simulink library "lib_fuel_cell"  (Simulink 4.00)
undefined symbols (not defined in the file or in its folder): air_cp, amb_tmp, cell_const_F, cell_const_g, cell_const_jo, cell_const_LHV_H2, cell_const_Mair, cell_const_MH, cell_const_MW, cell_const_R2, cell_const_Voc, ex_gas_cp, fan_cool, fc_acc_mass, fc_act, fc_air_comp_map, fc_air_comp_pwr, fc_base_mass, fc_blower_rec_H2, fc_blowera, fc_c2i_th_cond, fc_c_init_tmp, fc_cell_area, fc_cell_const_eta1, fc_cell_const_eta_DCDC, fc_cell_const_etablow, fc_cell_const_etagen, fc_cell_const_etapump, fc_cell_const_ex, fc_cell_const_kw, fc_cell_const_Nrad, fc_cell_const_U, fc_cell_dim_A, fc_cell_dim_tm, fc_cell_num, fc_cell_press_a, fc_cell_press_amb, fc_cell_press_an, fc_cell_press_blowa, fc_cell_press_blowr, fc_cell_press_c, fc_cell_press_hum, fc_cell_press_hyd, fc_cell_stack_dpipe, fc_cell_stack_dpipefc, fc_cell_stack_drad, fc_cell_stack_Lpipe, fc_cell_stack_Lpipefc, fc_cell_stack_Lrad, fc_cell_stack_N, fc_cell_stack_Pel, fc_cell_stoich_RHah, fc_cell_stoich_RHch, fc_cell_stoich_RHo, fc_cell_stoich_vH, fc_cell_stoich_vO, fc_cell_stoich_XON, fc_cell_temp_ah, fc_cell_temp_amb, fc_cell_temp_cell ... (+74)
libraries: fc_vt_lib x2, lib_fuel_cell x1
(part 1 of 5)
settings Model: LastModifiedBy=kharalds

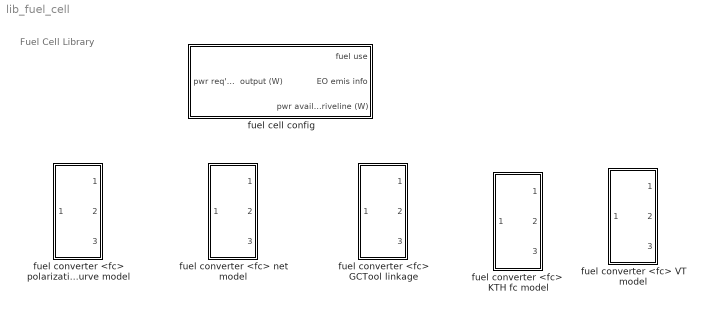
== system lib_fuel_cell ==
  note: Fuel Cell Library
  fuel cell config : Subsystem  BlockChoice=fuel converter <fc> net model
      settings: TemplateBlock=self  MemberBlocks="fuel converter <fc>  KTH fc model,fuel converter <fc> GCTool linkage,fuel converter <fc> VT model,fuel converter <fc> net model,fuel converter <fc> polarization curve model"  RTWFcnNameOpts=Auto  RTWFileNameOpts=Auto
  fuel converter <fc>  KTH fc model : Subsystem
      settings: RTWFcnNameOpts=Auto  RTWFileNameOpts=Auto
      mask Display: image(imread('bdi_fuelcell.jpg'))
  fuel converter <fc> GCTool linkage : Subsystem
      settings: RTWFcnNameOpts=Auto  RTWFileNameOpts=Auto
      mask Display: image(imread('bdi_fuelcell.jpg'))
  fuel converter <fc> VT model : Subsystem
      settings: RTWFcnNameOpts=Auto  RTWFileNameOpts=Auto
      mask Display: image(imread('bdi_fuelcell.jpg'))
  fuel converter <fc> net model : Subsystem
      settings: RTWFcnNameOpts=Auto  RTWFileNameOpts=Auto
      mask Display: image(imread('bdi_fuelcell.jpg'))
  fuel converter <fc> polarization curve model : Subsystem
      settings: RTWFcnNameOpts=Auto  RTWFileNameOpts=Auto
      mask Display: image(imread('bdi_fuelcell.jpg'))

== system lib_fuel_cell/fuel cell config ==
  pwr req'd at fc  output (W) : Inport  Port=1  LatchInput=off
  fuel converter <fc> net model : lib_fuel_cell/fuel converter <fc> net model
      link override fuel use and EO emis Fuel Cell/HOT engine maps /fuel (g//s): OutputValues=fc_fuel_map*fc_pwr_scale/fc_eff_scale
  fuel use : Outport  Port=1
  EO emis info : Outport  Port=2
  pwr avail. to driveline (W) : Outport  Port=3
  wires:
  pwr req'd at fc  output (W)/1 -> fuel converter <fc> net model/1
  fuel converter <fc> net model/1 -> fuel use/1
  fuel converter <fc> net model/2 -> EO emis info/1
  fuel converter <fc> net model/3 -> pwr avail. to driveline (W)/1

== system lib_fuel_cell/fuel converter <fc>  KTH fc model ==
  pwr req'd at fc  output (W) : Inport  Port=1  LatchInput=off
  Block NOTES : Subsystem
      settings: RTWFcnNameOpts=Auto  RTWFileNameOpts=Auto
      mask Display: disp('Block\nNOTES')
  Demux : Demux  Outputs=[1 4 1 1 1]  BusSelectionMode=off
  Demux1 : Demux  Outputs=[1 7 1]  BusSelectionMode=off
  Diagnostics : Subsystem
      settings: RTWFcnNameOpts=Auto  RTWFileNameOpts=Auto
  Mux1 : Mux  Inputs=7
  Temporary temperature : Constant  Value=[90 80 70 60]
  To Workspace2 : ToWorkspace  VariableName=fc_pwr_out_r  SampleTime=-1  SaveFormat=Array
  fuel cell  system <fc> : Subsystem
      settings: RTWFcnNameOpts=Auto  RTWFileNameOpts=Auto
  fuel use and EO emis Fuel Cell : Subsystem
      settings: RTWFcnNameOpts=Auto  RTWFileNameOpts=Auto
  fuel use : Outport  Port=1  InitialOutput=0
  EO emis info : Outport  Port=2  InitialOutput=0
  pwr avail. to driveline (W) : Outport  Port=3  InitialOutput=0
  tag scope: fc_pwr_out_a=global, fuel=global
  wires:
  fuel use and EO emis Fuel Cell/1(cum fuel  use (gal)) -> [fuel], fuel use/1
  fuel cell  system <fc>/1(power available (W) 1x1 emis info 7x1 fuel use 1x1) -> Demux1/1
  fuel use and EO emis Fuel Cell/3(Vv) -> Mux1/6
  fuel use and EO emis Fuel Cell/2("FC ON?, CO HC NOx PM mass flow exhaust exhaust temperature O2") -> Demux/1
  Demux1/1 -> pwr avail. to driveline (W)/1, [fc_pwr_out_a], fuel use and EO emis Fuel Cell/1(pwr (w))
  Demux1/2 -> fuel use and EO emis Fuel Cell/2(perf info)
  Demux1/3 -> fuel use and EO emis Fuel Cell/3(fuel use)
  pwr req'd at fc  output (W)/1 -> fuel cell  system <fc>/1(pwr req  (W)), To Workspace2/1
  fuel cell  system <fc>/2(system_characteristics) -> Diagnostics/1(In1)
  Temporary temperature/1 -> Mux1/7
  Mux1/1 -> EO emis info/1
  Demux/1 -> Mux1/1
  Demux/2 -> Mux1/2
  Demux/3 -> Mux1/3
  Demux/4 -> Mux1/4
  Demux/5 -> Mux1/5

== system lib_fuel_cell/fuel converter <fc> GCTool linkage ==
  pwr req'd at fc  output (W) : Inport  Port=1  LatchInput=off
  Block NOTES : Subsystem
      settings: RTWFcnNameOpts=Auto  RTWFileNameOpts=Auto
      mask Display: disp('Block\nNOTES')
  Constant : Constant  Value=fc_tstat
  Constant1 : Constant  Orientation=left  Value=0
  Constant3 : Constant  Value=fc_fuelcell_warmup_bool
  Constant4 : Constant  Orientation=left  Value=1
  Demux1 : Demux  Outputs=[1 7 1]  BusSelectionMode=off
  Mux : Mux  Inputs=2
      settings: DisplayOption=none
  Sum6 : Sum  Inputs=-+  SaturateOnIntegerOverflow=on
  Switch : Switch  Threshold=0
  Switch3 : Switch  Threshold=eps
  To Workspace2 : ToWorkspace  VariableName=fc_pwr_out_r  SampleTime=-1  SaveFormat=Array
  fuel cell  system <fc> : Subsystem
      settings: RTWFcnNameOpts=Auto  RTWFileNameOpts=Auto
  fuel use and EO emis Fuel Cell : Subsystem
      settings: RTWFcnNameOpts=Auto  RTWFileNameOpts=Auto
  gain : Gain  Gain=0.85  Multiplication=Element-wise(K.*u)  SaturateOnIntegerOverflow=on
  fuel use : Outport  Port=1  InitialOutput=0
  EO emis info : Outport  Port=2  InitialOutput=0
  pwr avail. to driveline (W) : Outport  Port=3  InitialOutput=0
  tag scope: fc_pwr_out_a=global, fuel=global
  wires:
  fuel use and EO emis Fuel Cell/1(cum fuel  use (gal)) -> [fuel], fuel use/1
  [coolant_temp] -> Sum6/2
  gain/1 -> Sum6/1
  Constant/1 -> gain/1
  Switch/1 -> [fc_pwr_out_a], pwr avail. to driveline (W)/1
  Switch3/1 -> Switch/2
  Sum6/1 -> Switch3/1
  Constant4/1 -> Switch3/3
  Constant3/1 -> Switch3/2
  Constant1/1 -> Switch/3
  pwr req'd at fc  output (W)/1 -> fuel cell  system <fc>/1(pwr req  (W)), To Workspace2/1
  fuel cell  system <fc>/1(power available (W) 1x1 emis info 7x1 fuel use 1x1) -> Demux1/1
  fuel use and EO emis Fuel Cell/3(Vv,Tfc) -> Mux/2
  fuel use and EO emis Fuel Cell/2("FC ON?, EOem, MFex, Tex, O2ex") -> Mux/1
  Mux/1 -> EO emis info/1
  Demux1/1 -> fuel use and EO emis Fuel Cell/1(pwr (w)), Switch/1
  Demux1/2 -> fuel use and EO emis Fuel Cell/2(perf info)
  Demux1/3 -> fuel use and EO emis Fuel Cell/3(fuel use)

== system lib_fuel_cell/fuel converter <fc> VT model ==
  note: May need to add enabled subsystem to top level (tm:8/12/02)
  pwr req'd at fc  output (W) : Inport  Port=1  LatchInput=off
  Block NOTES : Subsystem
      settings: RTWFcnNameOpts=Auto  RTWFileNameOpts=Auto
      mask Display: disp('Block\nNOTES')
  Fuel Cell Power System Model (S. Gurski - Virgina Tech) : Subsystem
      settings: RTWFcnNameOpts=Auto  RTWFileNameOpts=Auto
  Mux : Mux  Inputs=2
      settings: DisplayOption=none
  To Workspace2 : ToWorkspace  VariableName=fc_pwr_out_r  SampleTime=-1  SaveFormat=Array
  diagnostics : Subsystem
      settings: RTWFcnNameOpts=Auto  RTWFileNameOpts=Auto
  fuel use and EO emis Fuel Cell : Subsystem
      settings: RTWFcnNameOpts=Auto  RTWFileNameOpts=Auto
  fuel use : Outport  Port=1  InitialOutput=0
  EO emis info : Outport  Port=2  InitialOutput=0
  pwr avail. to driveline (W) : Outport  Port=3  InitialOutput=0
  tag scope: fc_pwr_out_a=global, fuel=global
  wires:
  Mux/1 -> EO emis info/1
  fuel use and EO emis Fuel Cell/2("FC ON?, EOem, MFex, Tex, O2ex") -> Mux/1
  fuel use and EO emis Fuel Cell/3(Vv,Tfc) -> Mux/2
  Fuel Cell Power System Model (S. Gurski - Virgina Tech)/1(Net Power Gen) -> fuel use and EO emis Fuel Cell/1(pwr (w)), pwr avail. to driveline (W)/1, [fc_pwr_out_a]
  pwr req'd at fc  output (W)/1 -> To Workspace2/1, Fuel Cell Power System Model (S. Gurski - Virgina Tech)/1(Net Power Request)
  fuel use and EO emis Fuel Cell/1(cum fuel  use (gal)) -> fuel use/1, [fuel]
  Fuel Cell Power System Model (S. Gurski - Virgina Tech)/2(system_characteristics) -> fuel use and EO emis Fuel Cell/2(system info), diagnostics/1(In1)

== system lib_fuel_cell/fuel converter <fc> net model ==
  pwr req'd at fc  output (W) : Inport  Port=1  LatchInput=off
  Block NOTES : Subsystem
      settings: RTWFcnNameOpts=Auto  RTWFileNameOpts=Auto
      mask Display: disp('Block\nNOTES')
  Constant : Constant  Value=fc_tstat
  Constant1 : Constant  Orientation=left  Value=0
  Constant3 : Constant  Value=fc_fuelcell_warmup_bool
  Constant4 : Constant  Orientation=left  Value=1
  Mux : Mux  Inputs=2
      settings: DisplayOption=none
  Sum6 : Sum  Inputs=-+  SaturateOnIntegerOverflow=on
  Switch : Switch  Threshold=0
  Switch3 : Switch  Threshold=eps
  To Workspace2 : ToWorkspace  VariableName=fc_pwr_out_r  SampleTime=-1  SaveFormat=Array
  fuel cell  system <fc> : Subsystem
      settings: RTWFcnNameOpts=Auto  RTWFileNameOpts=Auto
  fuel use and EO emis Fuel Cell : Subsystem
      settings: RTWFcnNameOpts=Auto  RTWFileNameOpts=Auto
  gain : Gain  Gain=0.85  Multiplication=Element-wise(K.*u)  SaturateOnIntegerOverflow=on
  fuel use : Outport  Port=1  InitialOutput=0
  EO emis info : Outport  Port=2  InitialOutput=0
  pwr avail. to driveline (W) : Outport  Port=3  InitialOutput=0
  tag scope: fc_pwr_out_a=global, fuel=global
  wires:
  Mux/1 -> EO emis info/1
  fuel use and EO emis Fuel Cell/2("FC ON?, EOem, MFex, Tex, O2ex") -> Mux/1
  fuel use and EO emis Fuel Cell/3(Vv,Tfc) -> Mux/2
  fuel cell  system <fc>/1(power available (W) 1x1) -> fuel use and EO emis Fuel Cell/1(pwr (w)), Switch/1
  pwr req'd at fc  output (W)/1 -> To Workspace2/1, fuel cell  system <fc>/1(pwr req  (W))
  Constant1/1 -> Switch/3
  Constant3/1 -> Switch3/2
  Constant4/1 -> Switch3/3
  Sum6/1 -> Switch3/1
  Switch3/1 -> Switch/2
  Switch/1 -> pwr avail. to driveline (W)/1, [fc_pwr_out_a]
  Constant/1 -> gain/1
  gain/1 -> Sum6/1
  [coolant_temp] -> Sum6/2
  fuel use and EO emis Fuel Cell/1(cum fuel  use (gal)) -> fuel use/1, [fuel]

== system lib_fuel_cell/fuel converter <fc> polarization curve model ==
  pwr req'd at fc  output (W) : Inport  Port=1  LatchInput=off
  Block NOTES : Subsystem
      settings: RTWFcnNameOpts=Auto  RTWFileNameOpts=Auto
      mask Display: disp('Block\nNOTES')
  Constant : Constant  Value=fc_tstat
  Constant1 : Constant  Orientation=left  Value=0
  Constant3 : Constant  Value=fc_fuelcell_warmup_bool
  Constant4 : Constant  Orientation=left  Value=1
  Demux1 : Demux  Outputs=[1 1 6 1 1]  BusSelectionMode=off
  Mux : Mux  Inputs=2
      settings: DisplayOption=none
  Sum6 : Sum  Inputs=-+  SaturateOnIntegerOverflow=on
  Switch : Switch  Threshold=0
  Switch3 : Switch  Threshold=eps
  To Workspace2 : ToWorkspace  VariableName=fc_pwr_out_r  SampleTime=-1  SaveFormat=Array
  fuel cell  system <fc> : Subsystem
      settings: RTWFcnNameOpts=Auto  RTWFileNameOpts=Auto
  fuel use and EO emis Fuel Cell : Subsystem
      settings: RTWFcnNameOpts=Auto  RTWFileNameOpts=Auto
  gain : Gain  Gain=0.85  Multiplication=Element-wise(K.*u)  SaturateOnIntegerOverflow=on
  fuel use : Outport  Port=1  InitialOutput=0
  EO emis info : Outport  Port=2  InitialOutput=0
  pwr avail. to driveline (W) : Outport  Port=3  InitialOutput=0
  tag scope: fc_pwr_out_a=global, fuel=global
  wires:
  fuel use and EO emis Fuel Cell/1(cum fuel  use (gal)) -> [fuel], fuel use/1
  [coolant_temp] -> Sum6/2
  gain/1 -> Sum6/1
  Constant/1 -> gain/1
  Switch/1 -> [fc_pwr_out_a], pwr avail. to driveline (W)/1
  Switch3/1 -> Switch/2
  Sum6/1 -> Switch3/1
  Constant4/1 -> Switch3/3
  Constant3/1 -> Switch3/2
  Constant1/1 -> Switch/3
  pwr req'd at fc  output (W)/1 -> fuel cell  system <fc>/1(pwr req  (W)), To Workspace2/1
  fuel cell  system <fc>/1(power net (W) 1x1 power gross (W) 1x1 emis info 6x1 fuel use 1x1 Texh 1x1) -> Demux1/1
  fuel use and EO emis Fuel Cell/3(Vv,Tfc) -> Mux/2
  fuel use and EO emis Fuel Cell/2("FC ON?, EOem, MFex, Tex, O2ex") -> Mux/1
  Mux/1 -> EO emis info/1
  Demux1/5 -> fuel use and EO emis Fuel Cell/5(Texh)
  Demux1/4 -> fuel use and EO emis Fuel Cell/4(fuel use)
  Demux1/3 -> fuel use and EO emis Fuel Cell/3(perf info)
  Demux1/1 -> fuel use and EO emis Fuel Cell/1(pwr net(w)), Switch/1
  Demux1/2 -> fuel use and EO emis Fuel Cell/2(pwr gross(w)1)

== system lib_fuel_cell/fuel converter <fc>  KTH fc model/Block NOTES ==
  note: This block models the internal combustion engine, and includes inertia effects,
      | performance limits, accessory loads, and temperature transient effects on fuel
      | use, engine-out emissions, and catalyst efficiency.  There are 'leads' to the
      | engine controller here, which controller determines whether the engine is on.

== system lib_fuel_cell/fuel converter <fc>  KTH fc model/Diagnostics ==
  In1 : Inport  Port=1  LatchInput=off
  Demux : Demux  Outputs=22  BusSelectionMode=off
  Terminator : Terminator
  Terminator1 : Terminator
  Terminator2 : Terminator
  To Workspace : ToWorkspace  VariableName=fc_net_pwr_req  SampleTime=-1  SaveFormat=Array
  To Workspace1 : ToWorkspace  VariableName=fc_net_pwr_gen  SampleTime=-1  SaveFormat=Array
  To Workspace10 : ToWorkspace  VariableName=fc_eta_fcsyst  SampleTime=-1  SaveFormat=Array
  To Workspace11 : ToWorkspace  VariableName=fc_gross_pwr  SampleTime=-1  SaveFormat=Array
  To Workspace13 : ToWorkspace  VariableName=fc_mdot_air  SampleTime=-1  SaveFormat=Array
  To Workspace14 : ToWorkspace  VariableName=w  SampleTime=-1  SaveFormat=Array
  To Workspace15 : ToWorkspace  VariableName=Qwc  SampleTime=-1  SaveFormat=Array
  To Workspace16 : ToWorkspace  VariableName=Qwa  SampleTime=-1  SaveFormat=Array
  To Workspace17 : ToWorkspace  VariableName=diff  SampleTime=-1  SaveFormat=Array
  To Workspace18 : ToWorkspace  VariableName=Qwtot  SampleTime=-1  SaveFormat=Array
  To Workspace19 : ToWorkspace  VariableName=Qevapc  SampleTime=-1  SaveFormat=Array
  To Workspace2 : ToWorkspace  VariableName=fc_auxiliary_pwr  SampleTime=-1  SaveFormat=Array
  To Workspace20 : ToWorkspace  VariableName=Qevapa  SampleTime=-1  SaveFormat=Array
  To Workspace21 : ToWorkspace  VariableName=Qhum  SampleTime=-1  SaveFormat=Array
  To Workspace3 : ToWorkspace  VariableName=fc_mdot_w_condc  SampleTime=-1  SaveFormat=Array
  To Workspace4 : ToWorkspace  VariableName=fc_current_density  SampleTime=-1  SaveFormat=Array
  To Workspace5 : ToWorkspace  VariableName=fc_mdot_H  SampleTime=-1  SaveFormat=Array
  To Workspace6 : ToWorkspace  VariableName=fc_mdot_w_conda  SampleTime=-1  SaveFormat=Array
  To Workspace9 : ToWorkspace  VariableName=fc_pwr_compressor  SampleTime=-1  SaveFormat=Array
  wires:
  In1/1 -> Demux/1
  Demux/1 -> To Workspace/1
  Demux/2 -> To Workspace1/1
  Demux/3 -> To Workspace2/1
  Demux/4 -> To Workspace3/1
  Demux/5 -> To Workspace4/1
  Demux/6 -> To Workspace5/1
  Demux/8 -> Terminator2/1
  Demux/10 -> To Workspace9/1
  Demux/11 -> To Workspace10/1
  Demux/12 -> To Workspace11/1
  Demux/13 -> Terminator1/1
  Demux/14 -> To Workspace13/1
  Demux/15 -> To Workspace14/1
  Demux/7 -> To Workspace6/1
  Demux/22 -> To Workspace21/1
  Demux/21 -> To Workspace20/1
  Demux/20 -> To Workspace19/1
  Demux/19 -> To Workspace18/1
  Demux/18 -> To Workspace16/1
  Demux/17 -> To Workspace15/1
  Demux/16 -> To Workspace17/1
  Demux/9 -> Terminator/1

== system lib_fuel_cell/fuel converter <fc>  KTH fc model/fuel cell  system <fc> ==
  pwr req  (W) : Inport  Port=1  LatchInput=off
  Block NOTES : Subsystem
      settings: RTWFcnNameOpts=Auto  RTWFileNameOpts=Auto
      mask Display: disp('Block\nNOTES')
  KTH fc model : Subsystem  TreatAsAtomicUnit=on
      settings: RTWFcnNameOpts=Auto  RTWFileNameOpts=Auto
  Mux2 : Mux  Inputs=[1 7 1]
      settings: DisplayOption=none
  power available (W) 1x1 emis info 7x1 fuel use 1x1 : Outport  Port=1  InitialOutput=0
  system_characteristics : Outport  Port=2  InitialOutput=0
  wires:
  [engine_on] -> KTH fc model/Enable
  Mux2/1 -> power available (W) 1x1 emis info 7x1 fuel use 1x1/1
  pwr req  (W)/1 -> KTH fc model/1(In1)
  KTH fc model/1(pwr avail. to driveline (W)) -> Mux2/1
  KTH fc model/2(Emissions info) -> Mux2/2
  KTH fc model/3(fuel use) -> Mux2/3
  KTH fc model/4(system characteristics) -> system_characteristics/1

== system lib_fuel_cell/fuel converter <fc>  KTH fc model/fuel use and EO emis Fuel Cell ==
  pwr (w) : Inport  Port=1  LatchInput=off
  perf info : Inport  Port=2  LatchInput=off
  fuel use : Inport  Port=3  LatchInput=off
  Block NOTES : Subsystem
      settings: RTWFcnNameOpts=Auto  RTWFileNameOpts=Auto
      mask Display: disp('Block\nNOTES')
  Demux1 : Demux  Outputs=7  BusSelectionMode=off
  Integrator : Integrator  ExternalReset=none  InitialConditionSource=internal  InitialCondition=0  LimitOutput=off  UpperSaturationLimit=inf  LowerSaturationLimit=-inf  ShowSaturationPort=off  ShowStatePort=off  AbsoluteTolerance=auto
  Mux1 : Mux  Inputs=4
      settings: DisplayOption=none
  Mux4 : Mux  Inputs=[1 4 1 1 1]
      settings: DisplayOption=none
  Terminator1 : Terminator
  To Workspace15 : ToWorkspace  VariableName=fc_fuel_rate  SampleTime=-1  SaveFormat=Array
  To Workspace8 : ToWorkspace  VariableName=fc_emis_eo  SampleTime=-1  SaveFormat=Array
  g/s-->gal/s : Gain  Gain=1/fc_fuel_den*61.02/231  Multiplication=Element-wise(K.*u)  SaturateOnIntegerOverflow=on
  cum fuel  use (gal) : Outport  Port=1  InitialOutput=0
  "FC ON?, CO HC NOx PM mass flow exhaust exhaust temperature O2" : Outport  Port=2  InitialOutput=0
  Vv : Outport  Port=3  InitialOutput=0
  wires:
  Demux1/7 -> Mux4/5
  Mux1/1 -> To Workspace8/1, Mux4/2
  g/s-->gal/s/1 -> Integrator/1
  Integrator/1 -> cum fuel  use (gal)/1
  Demux1/5 -> Mux4/3
  Demux1/6 -> Mux4/4
  pwr (w)/1 -> Terminator1/1
  perf info/1 -> Demux1/1
  Demux1/1 -> Mux1/1
  Demux1/2 -> Mux1/2
  Demux1/3 -> Mux1/3
  Demux1/4 -> Mux1/4
  fuel use/1 -> g/s-->gal/s/1, To Workspace15/1
  [v_prev] -> Vv/1
  [engine_on] -> Mux4/1
  Mux4/1 -> "FC ON?, CO HC NOx PM mass flow exhaust exhaust temperature O2"/1

== system lib_fuel_cell/fuel converter <fc> GCTool linkage/Block NOTES ==
  note: This block models the internal combustion engine, and includes inertia effects,
      | performance limits, accessory loads, and temperature transient effects on fuel
      | use, engine-out emissions, and catalyst efficiency.  There are 'leads' to the
      | engine controller here, which controller determines whether the engine is on.

== system lib_fuel_cell/fuel converter <fc> GCTool linkage/fuel cell  system <fc> ==
  pwr req  (W) : Inport  Port=1  LatchInput=off
  Block NOTES : Subsystem
      settings: RTWFcnNameOpts=Auto  RTWFileNameOpts=Auto
      mask Display: disp('Block\nNOTES')
  GCTool fuel cell model : Subsystem  TreatAsAtomicUnit=on
      settings: RTWFcnNameOpts=Auto  RTWFileNameOpts=Auto
  Mux2 : Mux  Inputs=[1 7 1]
      settings: DisplayOption=none
  power available (W) 1x1 emis info 7x1 fuel use 1x1 : Outport  Port=1  InitialOutput=0
  wires:
  pwr req  (W)/1 -> GCTool fuel cell model/1(net pwr req (W))
  Mux2/1 -> power available (W) 1x1 emis info 7x1 fuel use 1x1/1
  [engine_on] -> GCTool fuel cell model/Enable
  GCTool fuel cell model/1(net pwr out (W)) -> Mux2/1
  GCTool fuel cell model/2(emis info hc co nox pm MFexh Texh O2) -> Mux2/2
  GCTool fuel cell model/3(fuel use) -> Mux2/3

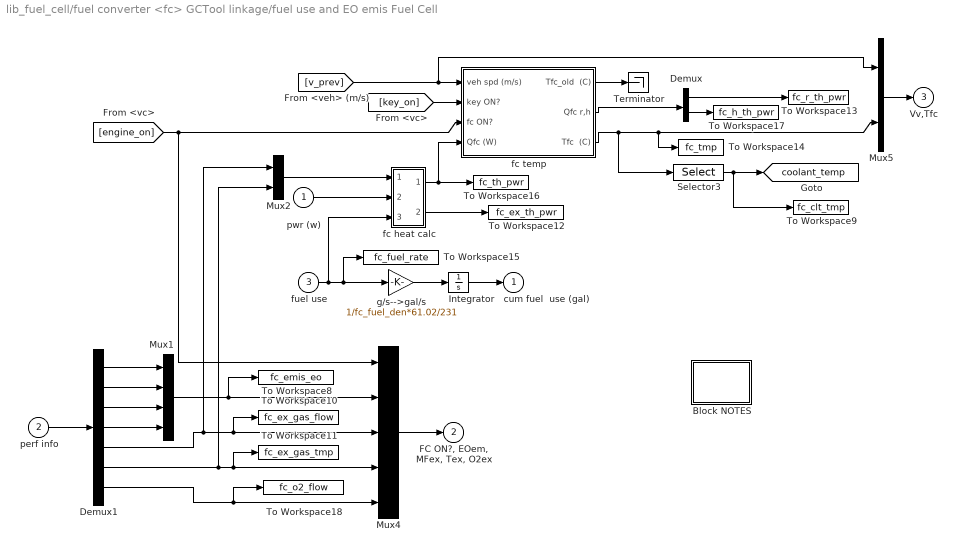
== system lib_fuel_cell/fuel converter <fc> GCTool linkage/fuel use and EO emis Fuel Cell ==
  pwr (w) : Inport  Port=1  LatchInput=off
  perf info : Inport  Port=2  LatchInput=off
  fuel use : Inport  Port=3  LatchInput=off
  Block NOTES : Subsystem
      settings: RTWFcnNameOpts=Auto  RTWFileNameOpts=Auto
      mask Display: disp('Block\nNOTES')
  Demux : Demux  Outputs=2  BusSelectionMode=off
  Demux1 : Demux  Outputs=7  BusSelectionMode=off
  Integrator : Integrator  ExternalReset=none  InitialConditionSource=internal  InitialCondition=0  LimitOutput=off  UpperSaturationLimit=inf  LowerSaturationLimit=-inf  ShowSaturationPort=off  ShowStatePort=off  AbsoluteTolerance=auto
  Mux1 : Mux  Inputs=4
      settings: DisplayOption=none
  Mux2 : Mux  Inputs=2
      settings: DisplayOption=none
  Mux4 : Mux  Inputs=[1 4 1 1 1]
      settings: DisplayOption=none
  Mux5 : Mux  Inputs=[1 4 ]
      settings: DisplayOption=none
  Selector3 : Selector  InputType=Vector  ElementSrc=Internal  Elements=2  RowSrc=Internal  Rows=1  ColumnSrc=Internal  Columns=1  InputPortWidth=4
  Terminator : Terminator
  To Workspace10 : ToWorkspace  VariableName=fc_ex_gas_flow  SampleTime=-1  SaveFormat=Array
  To Workspace11 : ToWorkspace  VariableName=fc_ex_gas_tmp  SampleTime=-1  SaveFormat=Array
  To Workspace12 : ToWorkspace  VariableName=fc_ex_th_pwr  SampleTime=-1  SaveFormat=Array
  To Workspace13 : ToWorkspace  VariableName=fc_r_th_pwr  SampleTime=-1  SaveFormat=Array
  To Workspace14 : ToWorkspace  VariableName=fc_tmp  SampleTime=-1  SaveFormat=Array
  To Workspace15 : ToWorkspace  VariableName=fc_fuel_rate  SampleTime=-1  SaveFormat=Array
  To Workspace16 : ToWorkspace  VariableName=fc_th_pwr  SampleTime=-1  SaveFormat=Array
  To Workspace17 : ToWorkspace  VariableName=fc_h_th_pwr  SampleTime=-1  SaveFormat=Array
  To Workspace18 : ToWorkspace  VariableName=fc_o2_flow  SampleTime=-1  SaveFormat=Array
  To Workspace8 : ToWorkspace  VariableName=fc_emis_eo  SampleTime=-1  SaveFormat=Array
  To Workspace9 : ToWorkspace  VariableName=fc_clt_tmp  SampleTime=-1  SaveFormat=Array
  fc heat calc : Subsystem
      settings: RTWFcnNameOpts=Auto  RTWFileNameOpts=Auto
  fc temp : Subsystem
      settings: RTWFcnNameOpts=Auto  RTWFileNameOpts=Auto
  g/s-->gal/s : Gain  Gain=1/fc_fuel_den*61.02/231  Multiplication=Element-wise(K.*u)  SaturateOnIntegerOverflow=on
  cum fuel  use (gal) : Outport  Port=1  InitialOutput=0
  "FC ON?, EOem, MFex, Tex, O2ex" : Outport  Port=2  InitialOutput=0
  Vv,Tfc : Outport  Port=3  InitialOutput=0
  tag scope: coolant_temp=global
  wires:
  Demux1/7 -> To Workspace18/1, Mux4/5
  Mux1/1 -> To Workspace8/1, Mux4/2
  g/s-->gal/s/1 -> Integrator/1
  Selector3/1 -> [coolant_temp], To Workspace9/1
  [engine_on] -> fc temp/3(fc ON?), Mux4/1
  Integrator/1 -> cum fuel  use (gal)/1
  Mux4/1 -> "FC ON?, EOem, MFex, Tex, O2ex"/1
  Demux1/5 -> To Workspace10/1, Mux4/3, Mux2/1
  Demux1/6 -> Mux4/4, To Workspace11/1, Mux2/2
  [key_on] -> fc temp/2(key ON?)
  Demux/2 -> To Workspace17/1
  Demux/1 -> To Workspace13/1
  fc temp/2(Qfc r,h) -> Demux/1
  fc temp/1(Tfc_old  (C)) -> Terminator/1
  fc temp/3(Tfc  (C)) -> Mux5/2, To Workspace14/1, Selector3/1
  [v_prev] -> fc temp/1(veh spd (m/s)), Mux5/1
  Mux5/1 -> Vv,Tfc/1
  pwr (w)/1 -> fc heat calc/2(In3)
  fc heat calc/2(Out1) -> To Workspace12/1
  perf info/1 -> Demux1/1
  Demux1/1 -> Mux1/1
  Demux1/2 -> Mux1/2
  Demux1/3 -> Mux1/3
  Demux1/4 -> Mux1/4
  Mux2/1 -> fc heat calc/1(In5)
  fc heat calc/1(Out2) -> fc temp/4(Qfc (W)), To Workspace16/1
  fuel use/1 -> g/s-->gal/s/1, To Workspace15/1, fc heat calc/3(In4)

== system lib_fuel_cell/fuel converter <fc> VT model/Block NOTES ==
  note: No block notes at this time.

== system lib_fuel_cell/fuel converter <fc> VT model/Fuel Cell Power System Model (S. Gurski - Virgina Tech) ==
  Net Power Request : Inport  Orientation=left  Port=1  LatchInput=off
  Algebraic Constraint1 : Subsystem  AncestorBlock=simulink3/Math/Algebraic Constraint  mask(Algebraic Constraint){z0=0.6}
      mask prompts: z0 "Initial guess:"
      mask help: Constrains input signal f(z) to zero and outputs an algebraic state z. This block outputs the value necessary to produce a zero at the input. The output must affect the input through some feedback path. Provide an initial guess of the output to improve algebraic loop solver efficiency.
      settings: RTWFcnNameOpts=Auto  RTWFileNameOpts=Auto
      mask Help:
      | This block outputs the value necessary to produce a zero at the input. The output must affect the input through some feedback path. This allows you to specify algebraic equations for index 1 differential/algebraic systems (DAE's).
      | 
      | By default, the initial guess is zero.  You can improve the efficiency of the algebraic loop solver by providing an initial guess that is close to the solution value.
      mask Display: disp('Solve\nf(z) = 0')
  Bus Creator : Subsystem
      settings: RTWFcnNameOpts=Auto  RTWFileNameOpts=Auto
  Constant1 : Constant  Value=fc_min_cell_volts
  Demux : Demux  Outputs=6  BusSelectionMode=off
  Demux1 : Demux  Outputs=6  BusSelectionMode=off
  Fuel Cell System : Subsystem  TreatAsAtomicUnit=on
      settings: RTWFcnNameOpts=Auto  RTWFileNameOpts=Auto
  Fuel Cell System - min voltage : Subsystem
      settings: RTWFcnNameOpts=Auto  RTWFileNameOpts=Auto
  If : If  NumInputs=2  IfExpression=u1 < u2  ShowElse=off
  Mux1 : Mux  Inputs=6
  Mux2 : Mux  Orientation=left  Inputs=6
  Sum2 : Sum  Inputs=|+-  SaturateOnIntegerOverflow=on
  Switch1 : Switch  Threshold=1
  Terminator : Terminator
  Water : Memory  Orientation=left  X0=0  InheritSampleTime=off
      settings: RTWStateStorageClass=Auto
  stack_temperature : Memory  Orientation=left  X0=fc_system_init_temp  InheritSampleTime=off
      settings: RTWStateStorageClass=Auto
  t_stack_coolant_in : Memory  Orientation=left  X0=fc_system_init_temp  InheritSampleTime=off
      settings: RTWStateStorageClass=Auto
  Net Power Gen : Outport  Port=1
  system_characteristics : Outport  Port=2
  wires:
  Demux/1 -> Net Power Gen/1
  Demux/2 -> stack_temperature/1
  Demux/4 -> t_stack_coolant_in/1
  Demux/5 -> Water/1
  t_stack_coolant_in/1 -> Mux2/2
  stack_temperature/1 -> Mux2/3
  Water/1 -> Mux2/4
  Bus Creator/1(system_characteristics) -> system_characteristics/1
  Demux/6 -> Bus Creator/1(In1)
  Net Power Request/1 -> Mux2/1
  Mux2/1 -> Demux1/1, Fuel Cell System/1(In1)
  Demux/3 -> Terminator/1
  [elevation] -> Mux2/5
  Constant1/1 -> Sum2/1
  Sum2/1 -> Algebraic Constraint1/1(f(z))
  Algebraic Constraint1/1(z) -> Fuel Cell System - min voltage/1(" Current Density Request")
  Fuel Cell System - min voltage/1(Net Power Gen) -> Mux1/1, If/2
  Fuel Cell System - min voltage/2(Stack Temperature) -> Mux1/2
  Fuel Cell System - min voltage/3(cell_voltage) -> Sum2/2, Mux1/3
  Fuel Cell System - min voltage/4(t_stack_coolant_in) -> Mux1/4
  Fuel Cell System - min voltage/5(waterbalance) -> Mux1/5
  Demux1/2 -> Fuel Cell System - min voltage/2(t_stack_coolant_in1)
  Demux1/3 -> Fuel Cell System - min voltage/3(fc_stack_temperature)
  Demux1/4 -> Fuel Cell System - min voltage/4(water_balance_previous)
  Demux1/1 -> If/1
  If/1 -> Fuel Cell System/Action
  Fuel Cell System/1(Out1) -> Switch1/1
  Fuel Cell System/2(Out2) -> Switch1/2
  Mux1/1 -> Switch1/3
  Fuel Cell System - min voltage/6(system_characteristics) -> Mux1/6
  Demux1/5 -> Fuel Cell System - min voltage/5(elevation)
  Switch1/1 -> Demux/1
  [v_prev] -> Mux2/6
  Demux1/6 -> Fuel Cell System - min voltage/6(vehicle speed (m/s))

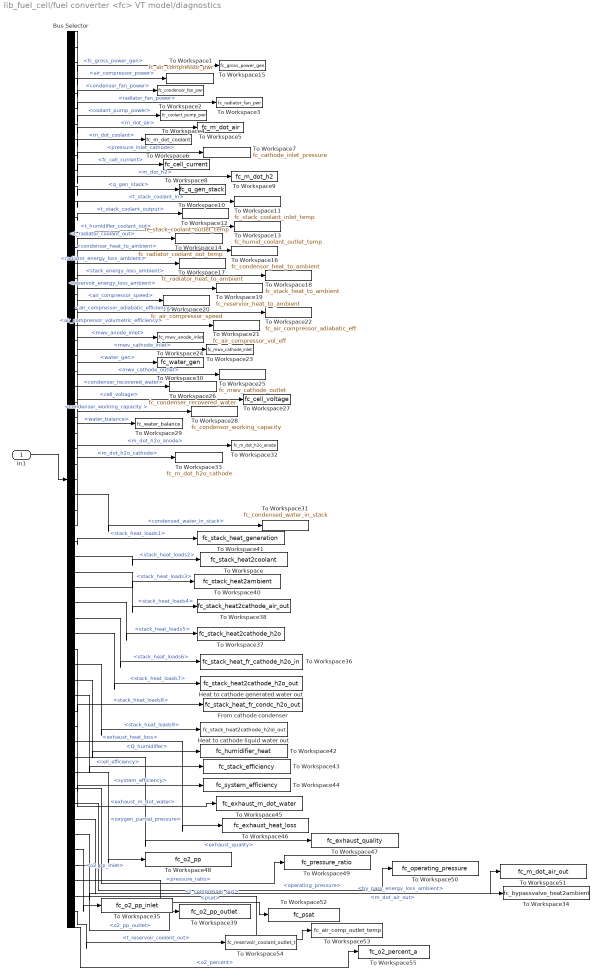
== system lib_fuel_cell/fuel converter <fc> VT model/diagnostics ==
  In1 : Inport  Port=1  LatchInput=off
  Bus Selector : BusSelector  OutputSignals=|  MuxedOutput=off
      | fc_gross_power_gen,air_compressor_power,condenser_fan_power,radiator_fan_power,coolant_pump_power,m_dot_air,m_dot_coolant,pressure_inlet_cathode,fc_cell_current,m_dot_h2,q_gen_stack,t_stack_coolant_in,t_stack_coolant_output,t_humidifier_coolant_out,t_radiator_coolant_out,condenser_heat_to_ambient,radiator_energy_loss_ambient,stack_energy_loss_ambient,reservoir_energy_loss_ambient,air_compressor_speed,air_compressor_adiabatic_efficiency,air_compressor_volumetric_efficiency,mwv_anode_inlet,mwv_cathode_inlet,water_gen,mwv_cathode_outlet,condenser_recovered_water,cell_voltage,condenser_working_capacity
      | ,water_balance,condensed_water_in_stack,m_dot_h2o_anode,m_dot_h2o_cathode,stack_heat_loads1,stack_heat_loads2,stack_heat_loads3,stack_heat_loads4,stack_heat_loads5,stack_heat_loads6,stack_heat_loads7,stack_heat_loads8,stack_heat_loads9,Q_humidifier,cell_efficiency,system_efficiency,exhaust_m_dot_water,exhaust_heat_loss,exhaust_quality,oxygen_partial_pressure,pressure_ratio,operating_pressure,m_dot_air_out,by_pass_energy_loss_ambient,o2_pp_inlet,o2_pp_outlet,psat,t_compresser_out,t_reservoir_coolant_out,o2_percent
  From cathode condenser : ToWorkspace  VariableName=fc_stack_heat_fr_condc_h2o_out  SampleTime=-1  SaveFormat=Array
  Heat to cathode generated water out : ToWorkspace  VariableName=fc_stack_heat2cathode_h2o_out  SampleTime=-1  SaveFormat=Array
  Heat to cathode liquid water out : ToWorkspace  VariableName=fc_stack_heat2cathode_h2ol_out  SampleTime=-1  SaveFormat=Array
  To Workspace : ToWorkspace  VariableName=fc_stack_heat2coolant  SampleTime=-1  SaveFormat=Array
  To Workspace1 : ToWorkspace  VariableName=fc_air_compressor_pwr  SampleTime=-1  SaveFormat=Array
  To Workspace10 : ToWorkspace  VariableName=fc_q_gen_stack  SampleTime=-1  SaveFormat=Array
  To Workspace11 : ToWorkspace  VariableName=fc_stack_coolant_inlet_temp  SampleTime=-1  SaveFormat=Array
  To Workspace12 : ToWorkspace  VariableName=fc_stack_coolant_outlet_temp  SampleTime=-1  SaveFormat=Array
  To Workspace13 : ToWorkspace  VariableName=fc_humid_coolant_outlet_temp  SampleTime=-1  SaveFormat=Array
  To Workspace14 : ToWorkspace  VariableName=fc_radiator_coolant_out_temp  SampleTime=-1  SaveFormat=Array
  To Workspace15 : ToWorkspace  VariableName=fc_gross_power_gen  SampleTime=-1  SaveFormat=Array
  To Workspace16 : ToWorkspace  VariableName=fc_condensor_heat_to_ambient  SampleTime=-1  SaveFormat=Array
  To Workspace17 : ToWorkspace  VariableName=fc_radiator_heat_to_ambient  SampleTime=-1  SaveFormat=Array
  To Workspace18 : ToWorkspace  VariableName=fc_stack_heat_to_ambient  SampleTime=-1  SaveFormat=Array
  To Workspace19 : ToWorkspace  VariableName=fc_reservior_heat_to_ambient  SampleTime=-1  SaveFormat=Array
  To Workspace2 : ToWorkspace  VariableName=fc_condensor_fan_pwr  SampleTime=-1  SaveFormat=Array
  To Workspace20 : ToWorkspace  VariableName=fc_air_compressor_speed  SampleTime=-1  SaveFormat=Array
  To Workspace21 : ToWorkspace  VariableName=fc_air_compressor_vol_eff  SampleTime=-1  SaveFormat=Array
  To Workspace22 : ToWorkspace  VariableName=fc_air_compressor_adiabatic_eff  SampleTime=-1  SaveFormat=Array
  To Workspace23 : ToWorkspace  VariableName=fc_mwv_cathode_inlet  SampleTime=-1  SaveFormat=Array
  To Workspace24 : ToWorkspace  VariableName=fc_mwv_anode_inlet  SampleTime=-1  SaveFormat=Array
  To Workspace25 : ToWorkspace  VariableName=fc_mwv_cathode_outlet  SampleTime=-1  SaveFormat=Array
  To Workspace26 : ToWorkspace  VariableName=fc_condenser_recovered_water  SampleTime=-1  SaveFormat=Array
  To Workspace27 : ToWorkspace  VariableName=fc_cell_voltage  SampleTime=-1  SaveFormat=Array
  To Workspace28 : ToWorkspace  VariableName=fc_condensor_working_capacity  SampleTime=-1  SaveFormat=Array
  To Workspace29 : ToWorkspace  VariableName=fc_water_balance  SampleTime=-1  SaveFormat=Array
  To Workspace3 : ToWorkspace  VariableName=fc_radiator_fan_pwr  SampleTime=-1  SaveFormat=Array
  To Workspace30 : ToWorkspace  VariableName=fc_water_gen  SampleTime=-1  SaveFormat=Array
  To Workspace31 : ToWorkspace  VariableName=fc_condensed_water_in_stack  SampleTime=-1  SaveFormat=Array
  To Workspace32 : ToWorkspace  VariableName=fc_m_dot_h2o_anode  SampleTime=-1  SaveFormat=Array
  To Workspace33 : ToWorkspace  VariableName=fc_m_dot_h2o_cathode  SampleTime=-1  SaveFormat=Array
  To Workspace34 : ToWorkspace  VariableName=fc_bypassvalve_heat2ambient  SampleTime=-1  SaveFormat=Array
  To Workspace35 : ToWorkspace  VariableName=fc_o2_pp_inlet  SampleTime=-1  SaveFormat=Array
  To Workspace36 : ToWorkspace  VariableName=fc_stack_heat_fr_cathode_h2o_in  SampleTime=-1  SaveFormat=Array
  To Workspace37 : ToWorkspace  VariableName=fc_stack_heat2cathode_h2o  SampleTime=-1  SaveFormat=Array
  To Workspace38 : ToWorkspace  VariableName=fc_stack_heat2cathode_air_out  SampleTime=-1  SaveFormat=Array
  To Workspace39 : ToWorkspace  VariableName=fc_o2_pp_outlet  SampleTime=-1  SaveFormat=Array
  To Workspace4 : ToWorkspace  VariableName=fc_coolant_pump_pwr  SampleTime=-1  SaveFormat=Array
  To Workspace40 : ToWorkspace  VariableName=fc_stack_heat2ambient  SampleTime=-1  SaveFormat=Array
  To Workspace41 : ToWorkspace  VariableName=fc_stack_heat_generation  SampleTime=-1  SaveFormat=Array
  To Workspace42 : ToWorkspace  VariableName=fc_humidifier_heat  SampleTime=-1  SaveFormat=Array
  To Workspace43 : ToWorkspace  VariableName=fc_stack_efficiency  SampleTime=-1  SaveFormat=Array
  To Workspace44 : ToWorkspace  VariableName=fc_system_efficiency  SampleTime=-1  SaveFormat=Array
  To Workspace45 : ToWorkspace  VariableName=fc_exhaust_m_dot_water  SampleTime=-1  SaveFormat=Array
  To Workspace46 : ToWorkspace  VariableName=fc_exhaust_heat_loss  SampleTime=-1  SaveFormat=Array
  To Workspace47 : ToWorkspace  VariableName=fc_exhaust_quality  SampleTime=-1  SaveFormat=Array
  To Workspace48 : ToWorkspace  VariableName=fc_o2_pp  SampleTime=-1  SaveFormat=Array
  To Workspace49 : ToWorkspace  VariableName=fc_pressure_ratio  SampleTime=-1  SaveFormat=Array
  To Workspace5 : ToWorkspace  VariableName=fc_m_dot_air  SampleTime=-1  SaveFormat=Array
  To Workspace50 : ToWorkspace  VariableName=fc_operating_pressure  SampleTime=-1  SaveFormat=Array
  To Workspace51 : ToWorkspace  VariableName=fc_m_dot_air_out  SampleTime=-1  SaveFormat=Array
  To Workspace52 : ToWorkspace  VariableName=fc_psat  SampleTime=-1  SaveFormat=Array
  To Workspace53 : ToWorkspace  VariableName=fc_air_comp_outlet_temp  SampleTime=-1  SaveFormat=Array
  To Workspace54 : ToWorkspace  VariableName=fc_reservoir_coolant_outlet_t  SampleTime=-1  SaveFormat=Array
  To Workspace55 : ToWorkspace  VariableName=fc_o2_percent_a  SampleTime=-1  SaveFormat=Array
  To Workspace6 : ToWorkspace  VariableName=fc_m_dot_coolant  SampleTime=-1  SaveFormat=Array
  To Workspace7 : ToWorkspace  VariableName=fc_cathode_inlet_pressure  SampleTime=-1  SaveFormat=Array
  To Workspace8 : ToWorkspace  VariableName=fc_cell_current  SampleTime=-1  SaveFormat=Array
  To Workspace9 : ToWorkspace  VariableName=fc_m_dot_h2  SampleTime=-1  SaveFormat=Array
  wires:
  In1/1 -> Bus Selector/1
  Bus Selector/1 -> To Workspace15/1  "<fc_gross_power_gen>"
  Bus Selector/2 -> To Workspace1/1  "<air_compressor_power>"
  Bus Selector/30 -> To Workspace29/1  "<water_balance>"
  Bus Selector/29 -> To Workspace28/1  "<condenser_working_capacity >"
  Bus Selector/28 -> To Workspace27/1  "<cell_voltage>"
  Bus Selector/27 -> To Workspace26/1  "<condenser_recovered_water>"
  Bus Selector/26 -> To Workspace25/1  "<mwv_cathode_outlet>"
  Bus Selector/25 -> To Workspace30/1  "<water_gen>"
  Bus Selector/24 -> To Workspace23/1  "<mwv_cathode_inlet>"
  Bus Selector/23 -> To Workspace24/1  "<mwv_anode_inlet>"
  Bus Selector/22 -> To Workspace21/1  "<air_compressor_volumetric_efficiency>"
  Bus Selector/21 -> To Workspace22/1  "<air_compressor_adiabatic_efficiency>"
  Bus Selector/20 -> To Workspace20/1  "<air_compressor_speed>"
  Bus Selector/19 -> To Workspace19/1  "<reservoir_energy_loss_ambient>"
  Bus Selector/18 -> To Workspace18/1  "<stack_energy_loss_ambient>"
  Bus Selector/17 -> To Workspace17/1  "<radiator_energy_loss_ambient>"
  Bus Selector/16 -> To Workspace16/1  "<condenser_heat_to_ambient>"
  Bus Selector/15 -> To Workspace14/1  "<t_radiator_coolant_out>"
  Bus Selector/14 -> To Workspace13/1  "<t_humidifier_coolant_out>"
  Bus Selector/13 -> To Workspace12/1  "<t_stack_coolant_output>"
  Bus Selector/12 -> To Workspace11/1  "<t_stack_coolant_in>"
  Bus Selector/11 -> To Workspace10/1  "<q_gen_stack>"
  Bus Selector/10 -> To Workspace9/1  "<m_dot_h2>"
  Bus Selector/9 -> To Workspace8/1  "<fc_cell_current>"
  Bus Selector/8 -> To Workspace7/1  "<pressure_inlet_cathode>"
  Bus Selector/7 -> To Workspace6/1  "<m_dot_coolant>"
  Bus Selector/6 -> To Workspace5/1  "<m_dot_air>"
  Bus Selector/5 -> To Workspace4/1  "<coolant_pump_power>"
  Bus Selector/4 -> To Workspace3/1  "<radiator_fan_power>"
  Bus Selector/3 -> To Workspace2/1  "<condenser_fan_power>"
  Bus Selector/31 -> To Workspace31/1  "<condensed_water_in_stack>"
  Bus Selector/32 -> To Workspace32/1  "<m_dot_h2o_anode>"
  Bus Selector/33 -> To Workspace33/1  "<m_dot_h2o_cathode>"
  Bus Selector/34 -> To Workspace41/1  "<stack_heat_loads1>"
  Bus Selector/35 -> To Workspace/1  "<stack_heat_loads2>"
  Bus Selector/36 -> To Workspace40/1  "<stack_heat_loads3>"
  Bus Selector/37 -> To Workspace38/1  "<stack_heat_loads4>"
  Bus Selector/38 -> To Workspace37/1  "<stack_heat_loads5>"
  Bus Selector/39 -> To Workspace36/1  "<stack_heat_loads6>"
  Bus Selector/40 -> Heat to cathode generated water out/1  "<stack_heat_loads7>"
  Bus Selector/41 -> From cathode condenser/1  "<stack_heat_loads8>"
  Bus Selector/42 -> Heat to cathode liquid water out/1  "<stack_heat_loads9>"
  Bus Selector/43 -> To Workspace42/1  "<Q_humidifier>"
  Bus Selector/44 -> To Workspace43/1  "<cell_efficiency>"
  Bus Selector/45 -> To Workspace44/1  "<system_efficiency>"
  Bus Selector/48 -> To Workspace47/1  "<exhaust_quality>"
  Bus Selector/47 -> To Workspace46/1  "<exhaust_heat_loss>"
  Bus Selector/46 -> To Workspace45/1  "<exhaust_m_dot_water>"
  Bus Selector/49 -> To Workspace48/1  "<oxygen_partial_pressure>"
  Bus Selector/50 -> To Workspace49/1  "<pressure_ratio>"
  Bus Selector/51 -> To Workspace50/1  "<operating_pressure>"
  Bus Selector/52 -> To Workspace51/1  "<m_dot_air_out>"
  Bus Selector/53 -> To Workspace34/1  "<by_pass_energy_loss_ambient>"
  Bus Selector/54 -> To Workspace35/1  "<o2_pp_inlet>"
  Bus Selector/55 -> To Workspace39/1  "<o2_pp_outlet>"
  Bus Selector/56 -> To Workspace52/1  "<psat>"
  Bus Selector/57 -> To Workspace53/1  "<t_compresser_out>"
  Bus Selector/58 -> To Workspace54/1  "<t_reservoir_coolant_out>"
  Bus Selector/59 -> To Workspace55/1  "<o2_percent>"

== system lib_fuel_cell/fuel converter <fc> VT model/fuel use and EO emis Fuel Cell ==
  pwr (w) : Inport  Port=1  LatchInput=off
  system info : Inport  Port=2  LatchInput=off
  Block NOTES : Subsystem
      settings: RTWFcnNameOpts=Auto  RTWFileNameOpts=Auto
      mask Display: disp('Block\nNOTES')
  Bus Selector : BusSelector  OutputSignals=m_dot_h2,t_stack_coolant_output  MuxedOutput=off
  Ground : Ground
  Integrator : Integrator  ExternalReset=none  InitialConditionSource=internal  InitialCondition=0  LimitOutput=off  UpperSaturationLimit=inf  LowerSaturationLimit=-inf  ShowSaturationPort=off  ShowStatePort=off  AbsoluteTolerance=auto
  Mux : Mux  Inputs=4
  Mux1 : Mux  Inputs=4
  Mux4 : Mux  Inputs=[1 4 1 1 1]
      settings: DisplayOption=none
  Mux5 : Mux  Inputs=[1 4 ]
      settings: DisplayOption=none
  Selector3 : Selector  InputType=Vector  ElementSrc=Internal  Elements=2  RowSrc=Internal  Rows=1  ColumnSrc=Internal  Columns=1  InputPortWidth=4
  Terminator1 : Terminator
  To Workspace14 : ToWorkspace  VariableName=fc_tmp  SampleTime=-1  SaveFormat=Array
  To Workspace15 : ToWorkspace  VariableName=fc_fuel_rate  SampleTime=-1  SaveFormat=Array
  To Workspace8 : ToWorkspace  VariableName=fc_emis_eo  SampleTime=-1  SaveFormat=Array
  To Workspace9 : ToWorkspace  VariableName=fc_clt_tmp  SampleTime=-1  SaveFormat=Array
  g/s-->gal/s : Gain  Gain=1/fc_fuel_den*61.02/231  Multiplication=Element-wise(K.*u)  SaturateOnIntegerOverflow=on
  kg/s-->g/s : Gain  Gain=1000  Multiplication=Element-wise(K.*u)  SaturateOnIntegerOverflow=on
  cum fuel  use (gal) : Outport  Port=1  InitialOutput=0
  "FC ON?, EOem, MFex, Tex, O2ex" : Outport  Port=2  InitialOutput=0
  Vv,Tfc : Outport  Port=3  InitialOutput=0
  tag scope: coolant_temp=global
  wires:
  Bus Selector/1 -> kg/s-->g/s/1  "<m_dot_h2>"
  Mux/1 -> To Workspace8/1, Mux4/2
  Ground/1 -> Mux/4, Mux/2, Mux/1, Mux1/4, Mux1/3, Mux1/1, Mux/3, Mux4/3, Mux4/4, Mux4/5
  g/s-->gal/s/1 -> Integrator/1
  [engine_on] -> Mux4/1
  Integrator/1 -> cum fuel  use (gal)/1
  Mux4/1 -> "FC ON?, EOem, MFex, Tex, O2ex"/1
  Mux1/1 -> Selector3/1, To Workspace14/1, Mux5/2
  [v_prev] -> Mux5/1
  Mux5/1 -> Vv,Tfc/1
  pwr (w)/1 -> Terminator1/1
  system info/1 -> Bus Selector/1
  kg/s-->g/s/1 -> To Workspace15/1, g/s-->gal/s/1
  Selector3/1 -> To Workspace9/1, [coolant_temp]
  Bus Selector/2 -> Mux1/2  "<t_stack_coolant_output>"

== system lib_fuel_cell/fuel converter <fc> net model/Block NOTES ==
  note: This block models the internal combustion engine, and includes inertia effects,
      | performance limits, accessory loads, and temperature transient effects on fuel
      | use, engine-out emissions, and catalyst efficiency.  There are 'leads' to the
      | engine controller here, which controller determines whether the engine is on.

== system lib_fuel_cell/fuel converter <fc> net model/fuel cell  system <fc> ==
  pwr req  (W) : Inport  Port=1  LatchInput=off
  Block NOTES : Subsystem
      settings: RTWFcnNameOpts=Auto  RTWFileNameOpts=Auto
      mask Display: disp('Block\nNOTES')
  pwr vs. eff  fuel cell model : Subsystem  TreatAsAtomicUnit=on
      settings: RTWFcnNameOpts=Auto  RTWFileNameOpts=Auto
  power available (W) 1x1 : Outport  Port=1  InitialOutput=0
  wires:
  pwr req  (W)/1 -> pwr vs. eff  fuel cell model/1(net pwr req (W))
  [engine_on] -> pwr vs. eff  fuel cell model/Enable
  pwr vs. eff  fuel cell model/1(net pwr avail (W)) -> power available (W) 1x1/1

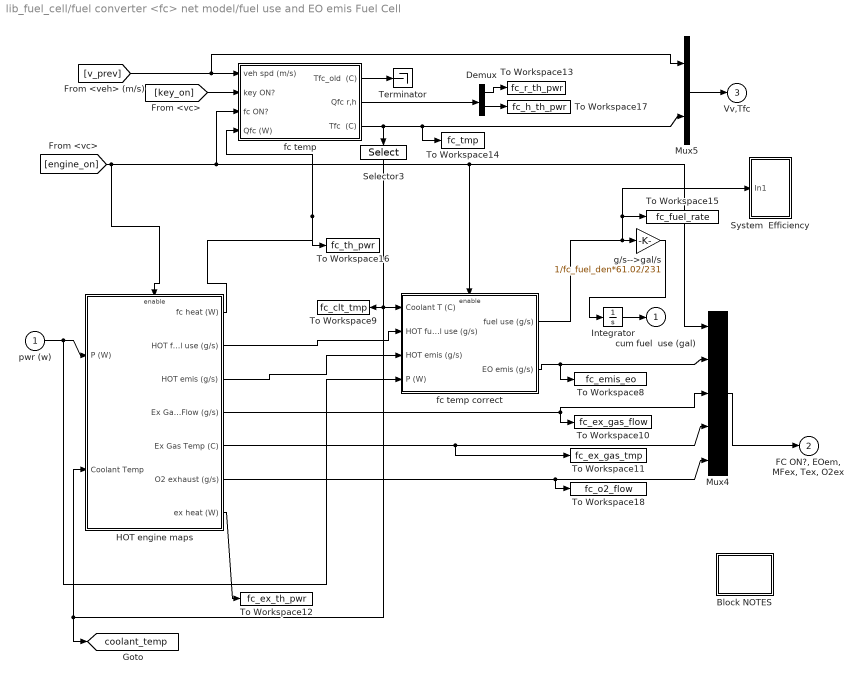
== system lib_fuel_cell/fuel converter <fc> net model/fuel use and EO emis Fuel Cell ==
  pwr (w) : Inport  Port=1  LatchInput=off
  Block NOTES : Subsystem
      settings: RTWFcnNameOpts=Auto  RTWFileNameOpts=Auto
      mask Display: disp('Block\nNOTES')
  Demux : Demux  Outputs=2  BusSelectionMode=off
  "HOT engine maps " : Subsystem  TreatAsAtomicUnit=on
      settings: RTWFcnNameOpts=Auto  RTWFileNameOpts=Auto
  Integrator : Integrator  ExternalReset=none  InitialConditionSource=internal  InitialCondition=0  LimitOutput=off  UpperSaturationLimit=inf  LowerSaturationLimit=-inf  ShowSaturationPort=off  ShowStatePort=off  AbsoluteTolerance=auto
  Mux4 : Mux  Inputs=[1 4 1 1 1]
      settings: DisplayOption=none
  Mux5 : Mux  Inputs=[1 4 ]
      settings: DisplayOption=none
  Selector3 : Selector  Orientation=down  InputType=Vector  ElementSrc=Internal  Elements=2  RowSrc=Internal  Rows=1  ColumnSrc=Internal  Columns=1  InputPortWidth=4
  System  Efficiency : Subsystem
      settings: RTWFcnNameOpts=Auto  RTWFileNameOpts=Auto
  Terminator : Terminator
  To Workspace10 : ToWorkspace  VariableName=fc_ex_gas_flow  SampleTime=-1  SaveFormat=Array
  To Workspace11 : ToWorkspace  VariableName=fc_ex_gas_tmp  SampleTime=-1  SaveFormat=Array
  To Workspace12 : ToWorkspace  VariableName=fc_ex_th_pwr  SampleTime=-1  SaveFormat=Array
  To Workspace13 : ToWorkspace  VariableName=fc_r_th_pwr  SampleTime=-1  SaveFormat=Array
  To Workspace14 : ToWorkspace  VariableName=fc_tmp  SampleTime=-1  SaveFormat=Array
  To Workspace15 : ToWorkspace  VariableName=fc_fuel_rate  SampleTime=-1  SaveFormat=Array
  To Workspace16 : ToWorkspace  VariableName=fc_th_pwr  SampleTime=-1  SaveFormat=Array
  To Workspace17 : ToWorkspace  VariableName=fc_h_th_pwr  SampleTime=-1  SaveFormat=Array
  To Workspace18 : ToWorkspace  VariableName=fc_o2_flow  SampleTime=-1  SaveFormat=Array
  To Workspace8 : ToWorkspace  VariableName=fc_emis_eo  SampleTime=-1  SaveFormat=Array
  To Workspace9 : ToWorkspace  VariableName=fc_clt_tmp  SampleTime=-1  SaveFormat=Array
  fc temp : Subsystem
      settings: RTWFcnNameOpts=Auto  RTWFileNameOpts=Auto
  fc temp correct : Subsystem  TreatAsAtomicUnit=on
      settings: RTWFcnNameOpts=Auto  RTWFileNameOpts=Auto
  g/s-->gal/s : Gain  Gain=1/fc_fuel_den*61.02/231  Multiplication=Element-wise(K.*u)  SaturateOnIntegerOverflow=on
  cum fuel  use (gal) : Outport  Port=1  InitialOutput=0
  "FC ON?, EOem, MFex, Tex, O2ex" : Outport  Port=2  InitialOutput=0
  Vv,Tfc : Outport  Port=3  InitialOutput=0
  tag scope: coolant_temp=global
  wires:
  "HOT engine maps "/6(O2 exhaust (g/s)) -> To Workspace18/1, Mux4/5
  fc temp correct/1(fuel use (g/s)) -> g/s-->gal/s/1, To Workspace15/1, System  Efficiency/1(In1)
  "HOT engine maps "/2(HOT fuel use (g/s)) -> fc temp correct/2(HOT fuel use (g/s))
  fc temp correct/2(EO emis (g/s)) -> To Workspace8/1, Mux4/2
  "HOT engine maps "/7(ex heat (W)) -> To Workspace12/1
  g/s-->gal/s/1 -> Integrator/1
  Selector3/1 -> [coolant_temp], "HOT engine maps "/2(Coolant Temp), To Workspace9/1, fc temp correct/1(Coolant T (C))
  [engine_on] -> fc temp/3(fc ON?), fc temp correct/Enable, Mux4/1, "HOT engine maps "/Enable
  Integrator/1 -> cum fuel  use (gal)/1
  Mux4/1 -> "FC ON?, EOem, MFex, Tex, O2ex"/1
  "HOT engine maps "/4(Ex Gas Flow (g/s)) -> To Workspace10/1, Mux4/3
  "HOT engine maps "/5(Ex Gas Temp (C)) -> Mux4/4, To Workspace11/1
  [key_on] -> fc temp/2(key ON?)
  Demux/2 -> To Workspace17/1
  Demux/1 -> To Workspace13/1
  fc temp/2(Qfc r,h) -> Demux/1
  fc temp/1(Tfc_old  (C)) -> Terminator/1
  fc temp/3(Tfc  (C)) -> Mux5/2, To Workspace14/1, Selector3/1
  [v_prev] -> fc temp/1(veh spd (m/s)), Mux5/1
  Mux5/1 -> Vv,Tfc/1
  "HOT engine maps "/3(HOT emis (g/s)) -> fc temp correct/3(HOT emis (g/s))
  pwr (w)/1 -> "HOT engine maps "/1(P (W)), fc temp correct/4(P (W))
  "HOT engine maps "/1(fc heat (W)) -> fc temp/4(Qfc (W)), To Workspace16/1

== system lib_fuel_cell/fuel converter <fc> polarization curve model/Block NOTES ==
  note: This block models the internal combustion engine, and includes inertia effects,
      | performance limits, accessory loads, and temperature transient effects on fuel
      | use, engine-out emissions, and catalyst efficiency.  There are 'leads' to the
      | engine controller here, which controller determines whether the engine is on.

== system lib_fuel_cell/fuel converter <fc> polarization curve model/fuel cell  system <fc> ==
  pwr req  (W) : Inport  Port=1  LatchInput=off
  Block NOTES : Subsystem
      settings: RTWFcnNameOpts=Auto  RTWFileNameOpts=Auto
      mask Display: disp('Block\nNOTES')
  Diagnostics : Subsystem
      settings: RTWFcnNameOpts=Auto  RTWFileNameOpts=Auto
  Mux2 : Mux  Inputs=[1 1 6 1 1]
      settings: DisplayOption=none
  polarization curve fuel cell model : Subsystem  TreatAsAtomicUnit=on
      settings: RTWFcnNameOpts=Auto  RTWFileNameOpts=Auto
  power net (W) 1x1 power gross (W) 1x1 emis info 6x1 fuel use 1x1 Texh 1x1 : Outport  Port=1  InitialOutput=0
  wires:
  pwr req  (W)/1 -> polarization curve fuel cell model/1(pwr req  (W))
  Mux2/1 -> power net (W) 1x1 power gross (W) 1x1 emis info 6x1 fuel use 1x1 Texh 1x1/1
  [engine_on] -> polarization curve fuel cell model/Enable
  polarization curve fuel cell model/1(pwr out a (W) Net) -> Mux2/1
  polarization curve fuel cell model/6(diagnostics) -> Diagnostics/1(In1)
  polarization curve fuel cell model/5("emis info Texh ") -> Mux2/5
  polarization curve fuel cell model/4(fuel use g/s) -> Mux2/4
  polarization curve fuel cell model/3(emis info hc co nox pm MFexh O2) -> Mux2/3
  polarization curve fuel cell model/2(pwr out a (W) Gross1) -> Mux2/2, Diagnostics/2(In2)
